simulink model "EMEAControls_BlockDiagram"  (R2016a)
settings: Solver=VariableStepAuto  StartTime=0.0  StopTime=10.0  RelTol=1e-3
undefined symbols (not defined in the file): ACTIVE, AIN03, AIN09, AIN13, AUX2, AUX2_FLOW_POT, BASE_ACTIVE, CD_AUX4_CONTROL_NEUTRAL, CD_AUX4_CRACKPOINT_CURRENT, CD_AUX4_MAX_FLOW_CURRENT, DIN08, DIN09, ENGINE_CRANKING, INIT_NORMAL, LEFT_HANDLE_BUTTON, LEFT_HANDLE_POT, MODE_AUX2_AUX4, MODE_AUX4_AUX2, MODE_AUX4_OFFSET, MODE_OFFSET_AUX4, MXSEC_AUX4_FLOW, NEUTRAL, OFFSET_SWITCH, RIGHT_HANDLE_POT, ROD_ACTIVE, SELECT_LEFT, SELECT_NEUTRAL, SELECT_RIGHT, SOC_LEFT, SOC_RIGHT
libraries: simulink x4, MX_Library x2
settings Model: Creator=aliebel  LastModifiedBy=aliebel

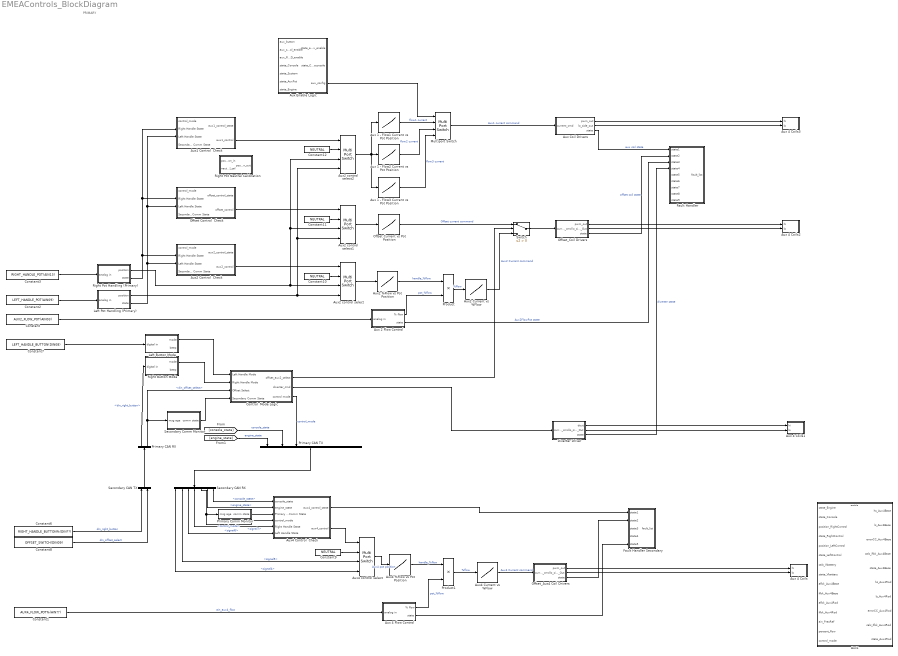
== system EMEAControls_BlockDiagram ==
  note: PRIMARY
  Aux 1 - Flow1 Current vs Pot Position : Lookup_n-D  NumberOfTableDimensions=1  BreakpointsForDimension1=[-5:5]  Table=tanh([-5:5])  InternalRulePriority=Speed  RndMeth=Simplest  InputSameDT=on
  Aux 1 - Flow2 Current vs Pot Position : Lookup_n-D  NumberOfTableDimensions=1  BreakpointsForDimension1=[-5:5]  Table=tanh([-5:5])  InternalRulePriority=Speed  RndMeth=Simplest  InputSameDT=on
  Aux 1 - Flow3 Current vs Pot Position : Lookup_n-D  NumberOfTableDimensions=1  BreakpointsForDimension1=[-5:5]  Table=tanh([-5:5])  InternalRulePriority=Speed  RndMeth=Simplest  InputSameDT=on
  Aux 2 Flow Control : Subsystem
  Aux 4 Coils : Subsystem
  Aux 4 Coils1 : Subsystem
  Aux 4 Coils2 : Subsystem
  Aux 4 Coils3 : Subsystem
  Aux 4 Flow Control : Subsystem
  Aux Coil Drivers : Subsystem
  Aux Enable Logic : Subsystem
  Aux1 : Subsystem
  Aux1 Control  Check : Subsystem
  Aux2 %Flow vs Pot Position : Lookup_n-D  NumberOfTableDimensions=1  BreakpointsForDimension1=[-5:5]  Table=tanh([-5:5])  InternalRulePriority=Speed  RndMeth=Simplest  InputSameDT=on
  Aux2 Current vs %Flow : Lookup_n-D  NumberOfTableDimensions=1  BreakpointsForDimension1=[-5:5]  Table=tanh([-5:5])  InternalRulePriority=Speed  RndMeth=Simplest  InputSameDT=on
  Aux2 Control  Check : Subsystem
  Aux2 control select : MultiPortSwitch
  Aux2 control select1 : MultiPortSwitch
  Aux2 control select2 : MultiPortSwitch
  Aux4 %Flow vs Pot Position : Lookup_n-D  NumberOfTableDimensions=1  BreakpointsForDimension1=[-5:5]  Table=tanh([-5:5])  InternalRulePriority=Speed  RndMeth=Simplest  InputSameDT=on
  Aux4 Current vs %Flow : Lookup_n-D  NumberOfTableDimensions=1  BreakpointsForDimension1=[-5:5]  Table=tanh([-5:5])  InternalRulePriority=Speed  RndMeth=Simplest  InputSameDT=on
  Aux4 Control  Check : Subsystem
  Aux4 control select : MultiPortSwitch
  Constant : Constant  Value=AUX2_FLOW_POT(AIN03)
  Constant1 : Constant  Value=AUX4_FLOW_POT%(AIN??)
  Constant{9..12} (4 alike) : Constant  Value=NEUTRAL
  Constant2 : Constant  Value=LEFT_HANDLE_POT(AIN09)
  Constant3 : Constant  Value=RIGHT_HANDLE_POT(AIN13)
  Constant6 : Constant  Value=RIGHT_HANDLE_BUTTON%(DIN??)
  Constant7 : Constant  Value=LEFT_HANDLE_BUTTON(DIN08)
  Constant8 : Constant  Value=OFFSET_SWITCH(DIN09)
  Control  Mode Logic : Subsystem
  Diverter Driver : Subsystem
  Fault Handler : Subsystem
  Fault Handler Secondary : Subsystem
  Left Button Mode : Subsystem
  Left Pot Handling (Primary) : Subsystem
  Multiport Switch : MultiPortSwitch
  Offset Current vs Pot Position : Lookup_n-D  NumberOfTableDimensions=1  BreakpointsForDimension1=[-5:5]  Table=tanh([-5:5])  InternalRulePriority=Speed  RndMeth=Simplest  InputSameDT=on
  Offset Control  Check : Subsystem
  Offset_Aux4 Coil Drivers : Subsystem
  Offset_Coil Drivers : Subsystem
  Primary CAN RX : BusSelector  OutputSignals=din_right_button,din_offset_select
  Primary CAN TX : BusCreator  Inputs=7
  Primary Comm Monitor : Subsystem
  Product : Product
  Product1 : Product
  Right Button Mode : Subsystem
  Right Pot Handling (Primary) : Subsystem
  Right Pot Neutral Calibration : Subsystem
  Secondary CAN RX : BusSelector  OutputSignals=signal4,signal5,signal6,signal7,control_mode,engine_state,console_state
  Secondary CAN TX : BusCreator  Inputs=2
  Secondary Comm Monitor : Subsystem
  Switch : Switch  Criteria=u2 > Threshold
  wires:
  Aux 1 - Flow1 Current vs Pot Position/1 -> Multiport Switch/2  "flow1 current"
  Multiport Switch/1 -> Aux Coil Drivers/1(current_cmd)  "Aux1 current command"
  Aux 1 - Flow2 Current vs Pot Position/1 -> Multiport Switch/3  "flow2 current"
  Aux 1 - Flow3 Current vs Pot Position/1 -> Multiport Switch/4  "flow3 current"
  Aux2 %Flow vs Pot Position/1 -> Product/1  "handle_%flow"
  Product/1 -> Aux2 Current vs %Flow/1  "%flow"
  Offset Current vs Pot Position/1 -> Switch/1  "Offset current command"
  Aux2 Current vs %Flow/1 -> Switch/3  "Aux2 Current command"
  Switch/1 -> Offset_Coil Drivers/1(current_cmd)
  Aux 2 Flow Control/1(% flow) -> Product/2  "pot_%flow"
  Aux4 %Flow vs Pot Position/1 -> Product1/1  "handle_%flow"
  Product1/1 -> Aux4 Current vs %Flow/1  "%flow"
  Aux4 Current vs %Flow/1 -> Offset_Aux4 Coil Drivers/1(current_cmd)  "Aux4 Current command"
  Aux 4 Flow Control/1(% flow) -> Product1/2  "pot_%flow"
  Aux Coil Drivers/3(state) -> Fault Handler/1(state1)  "aux coil state"
  Offset_Coil Drivers/3(state) -> Fault Handler/2(state2)  "offset coil state"
  Diverter Driver/3(state) -> Fault Handler/4(state4)  "diverter state"
  Aux 2 Flow Control/2(state) -> Fault Handler/3(state3)  "Aux2FlowPot state"
  Constant/1 -> Aux 2 Flow Control/1(analog in)
  Constant1/1 -> Aux 4 Flow Control/1(analog in)  "ain_aux4_flow"
  Primary CAN TX/1 -> Secondary CAN RX/1
  Secondary CAN TX/1 -> Primary CAN RX/1
  Constant7/1 -> Left Button Mode/1(digital in)
  Constant2/1 -> Left Pot Handling (Primary)/1(analog in)
  Constant3/1 -> Right Pot Handling (Primary)/1(analog in)
  Constant8/1 -> Secondary CAN TX/2  "din_offset_select"
  Constant6/1 -> Secondary CAN TX/1  "din_right_button"
  Primary Comm Monitor/1(comm state) -> Aux4 Control  Check/3(Primary Comm State)
  Secondary CAN RX/5 -> Primary Comm Monitor/1(msg age), Aux4 Control  Check/4(control_mode)  "<control_mode>"
  Aux4 Control  Check/1(aux4_control_state) -> Fault Handler Secondary/1(state1)
  Offset_Aux4 Coil Drivers/3(state) -> Fault Handler Secondary/2(state2)
  Aux4 Control  Check/2(aux4_control) -> Aux4 control select/1
  Constant9/1 -> Aux4 control select/2
  Aux4 control select/1 -> Aux4 %Flow vs Pot Position/1  "Aux4 pot position"
  Aux 4 Flow Control/2(state) -> Fault Handler Secondary/5(state5)
  Primary CAN RX/2 -> Control  Mode Logic/3(Offset Select), Secondary Comm Monitor/1(msg age)  "<din_offset_select>"
  Offset_Aux4 Coil Drivers/1(pwm_out) -> Aux 4 Coils/1("hi ")
  Offset_Aux4 Coil Drivers/2(lo_side_Out) -> Aux 4 Coils/2(lo)
  Primary CAN RX/1 -> Right Button Mode/1(digital in)  "<din_right_button>"
  Secondary Comm Monitor/1(comm state) -> Control  Mode Logic/4(Secondary Comm State)
  Right Button Mode/1(mode) -> Control  Mode Logic/2(Right Handle Mode)
  Left Button Mode/1(mode) -> Control  Mode Logic/1(Left Handle Mode)
  Control  Mode Logic/3(control mode) -> Primary CAN TX/3  "control_mode"
  Aux2 control select/1 -> Aux2 %Flow vs Pot Position/1
  Constant10/1 -> Aux2 control select/2
  Aux2 Control  Check/2(aux2_control) -> Aux2 control select/1
  Diverter Driver/1(dout) -> Aux 4 Coils1/1("hi ")
  Diverter Driver/2(lo_side_Out) -> Aux 4 Coils1/2(lo)
  Offset_Coil Drivers/1(pwm_out) -> Aux 4 Coils2/1("hi ")
  Offset_Coil Drivers/2(lo_side_Out) -> Aux 4 Coils2/2(lo)
  Aux Coil Drivers/1(pwm_out) -> Aux 4 Coils3/1("hi ")
  Aux Coil Drivers/2(lo_side_out) -> Aux 4 Coils3/2(lo)
  Constant11/1 -> Aux2 control select1/2
  Constant12/1 -> Aux2 control select2/2
  Aux2 control select2/1 -> Aux 1 - Flow1 Current vs Pot Position/1, Aux 1 - Flow3 Current vs Pot Position/1, Aux 1 - Flow2 Current vs Pot Position/1
  Aux2 control select1/1 -> Offset Current vs Pot Position/1
  Offset Control  Check/2(offset_control) -> Aux2 control select1/1
  Aux1 Control  Check/2(aux1_control) -> Aux2 control select2/1
  Left Pot Handling (Primary)/1(position) -> Aux2 control select2/4, Aux2 control select1/4, Aux2 control select/4
  Right Pot Handling (Primary)/1(position) -> Aux2 control select2/3, Aux2 control select1/3, Aux2 control select/3
  Right Pot Handling (Primary)/2(state) -> Offset Control  Check/2(Right Handle State), Aux1 Control  Check/2(Right Handle State), Aux2 Control  Check/2(Right Handle State)
  Left Pot Handling (Primary)/2(state) -> Aux1 Control  Check/3(Left Handle State), Offset Control  Check/3(Left Handle State), Aux2 Control  Check/3(Left Handle State)
  Control  Mode Logic/2(diverter_cmd) -> Diverter Driver/1(current_cmd)
  Control  Mode Logic/1(offset_aux2_select) -> Switch/2
  Aux Enable Logic/3(aux_config) -> Multiport Switch/1
  [console_state] -> Primary CAN TX/2  "console_state"
  [engine_state] -> Primary CAN TX/1  "engine_state"
  Secondary CAN RX/6 -> Aux4 Control  Check/2(engine_state)  "<engine_state>"
  Secondary CAN RX/7 -> Aux4 Control  Check/1(console_state)  "<console_state>"
  Secondary CAN RX/4 -> Aux4 Control  Check/5(Right Handle State)  "<signal7>"
  Secondary CAN RX/3 -> Aux4 Control  Check/6(Left Handle State)  "<signal6>"
  Secondary CAN RX/2 -> Aux4 control select/3  "<signal5>"
  Secondary CAN RX/1 -> Aux4 control select/4  "<signal4>"

== system EMEAControls_BlockDiagram/Aux 2 Flow Control ==
  analog in : Inport
  % flow : Outport
  state : Outport  Port=2
  wires:
  analog in/1 -> % flow/1

== system EMEAControls_BlockDiagram/Aux 4 Coils ==
  "hi " : Inport
  lo : Inport  Port=2

== system EMEAControls_BlockDiagram/Aux 4 Coils1 ==
  "hi " : Inport
  lo : Inport  Port=2

== system EMEAControls_BlockDiagram/Aux 4 Coils2 ==
  "hi " : Inport
  lo : Inport  Port=2

== system EMEAControls_BlockDiagram/Aux 4 Coils3 ==
  "hi " : Inport
  lo : Inport  Port=2

== system EMEAControls_BlockDiagram/Aux 4 Flow Control ==
  analog in : Inport
  % flow : Outport
  state : Outport  Port=2
  wires:
  analog in/1 -> % flow/1

== system EMEAControls_BlockDiagram/Aux Coil Drivers ==
  current_cmd : Inport
  pwm_out : Outport
  lo_side_out : Outport  Port=2
  state : Outport  Port=3
  wires:
  current_cmd/1 -> pwm_out/1

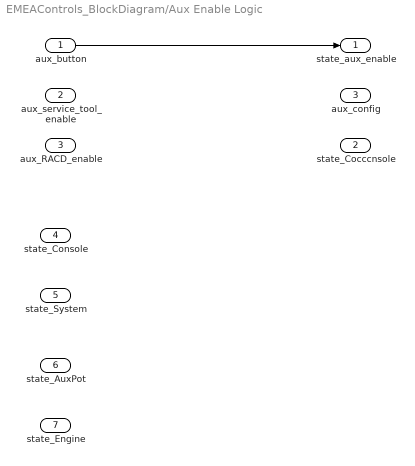
== system EMEAControls_BlockDiagram/Aux Enable Logic ==
  aux_button : Inport
  aux_service_tool_enable : Inport  Port=2
  aux_RACD_enable : Inport  Port=3
  state_Console : Inport  Port=4
  state_System : Inport  Port=5
  state_AuxPot : Inport  Port=6
  state_Engine : Inport  Port=7
  state_aux_enable : Outport
  state_Cocccnsole : Outport  Port=2
  aux_config : Outport  Port=3
  wires:
  aux_button/1 -> state_aux_enable/1

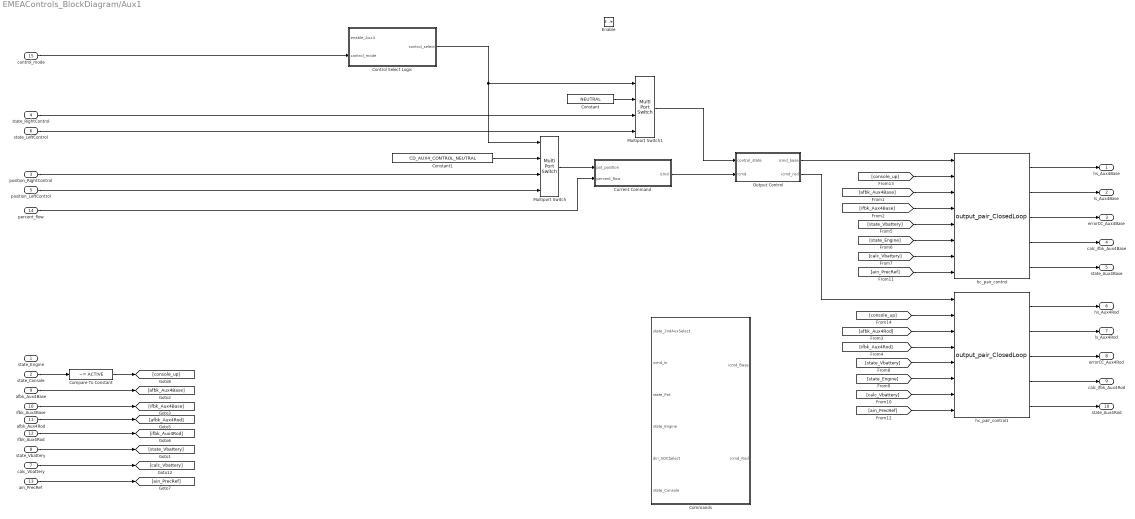
== system EMEAControls_BlockDiagram/Aux1 ==
  state_Engine : Inport
  state_Console : Inport  Port=2
  position_RightControl : Inport  Port=3
  state_RightControl : Inport  Port=4
  position_LeftControl : Inport  Port=5
  state_LeftControl : Inport  Port=6
  calc_Vbattery : Inport  Port=7
  state_Vbattery : Inport  Port=8
  afbk_Aux4Base : Inport  Port=9
  ifbk_Aux4Base : Inport  Port=10
  afbk_Aux4Rod : Inport  Port=11
  ifbk_Aux4Rod : Inport  Port=12
  ain_PrecRef : Inport  Port=13
  percent_flow : Inport  Port=14
  control_mode : Inport  Port=15
  Enable : EnablePort  StatesWhenEnabling=reset  PropagateVarSize=During execution
  Commands : Stateflow chart  TreatAsAtomicUnit=on
  Compare To Constant : simulink/Logic and Bit Operations/Compare To Constant  relop=~=  const=ACTIVE  OutDataTypeStr=boolean
  Constant : Constant  Value=NEUTRAL  OutDataTypeStr=uint8
  Constant1 : Constant  Value=CD_AUX4_CONTROL_NEUTRAL  OutDataTypeStr=uint8
  Control Select Logic : Truth Table  TreatAsAtomicUnit=on
  Current Command : Subsystem
  Multiport Switch : MultiPortSwitch
  Multiport Switch1 : MultiPortSwitch
  Output Control : Subsystem
  hc_pair_control : MX_Library/output_pair_ClosedLoop  AFBK_GAIN=CD_AUX4_AFBK_GAIN  IFBK_GAIN=CD_AUX4_IFBK_GAIN  OPEN_DB_CNT=CD_AUX4_DEBOUNCE_OPEN_CIRCUIT  STG_DB_CNT=CD_AUX4_DEBOUNCE_SHORT_TO_GROUND  OSTG_DB_CNT=CD_AUX4_DEBOUNCE_SHORT_TO_GROUND  STB_DB_CNT=CD_AUX4_DEBOUNCE_SHORT_TO_BATTERY  OC_DB_CNT=CD_AUX4_DEBOUNCE_OVERCURRENT  IFBK_MAX=CD_AUX4_OVERCURRENT  NZ_IFBK=CD_AUX4_NON_ZERO_CURRENT  NZ_DUTY=CD_AUX4_NON_ZERO_DUTY  KP=CD_AUX4_KP  KI=CD_AUX4_KI  BIDIRECTIONAL_CTRL=NON_FUNCTIONAL
  hc_pair_control1 : MX_Library/output_pair_ClosedLoop  AFBK_GAIN=CD_AUX4_AFBK_GAIN  IFBK_GAIN=CD_AUX4_IFBK_GAIN  OPEN_DB_CNT=CD_AUX4_DEBOUNCE_OPEN_CIRCUIT  STG_DB_CNT=CD_AUX4_DEBOUNCE_SHORT_TO_GROUND  OSTG_DB_CNT=CD_AUX4_DEBOUNCE_SHORT_TO_GROUND  STB_DB_CNT=CD_AUX4_DEBOUNCE_SHORT_TO_BATTERY  OC_DB_CNT=CD_AUX4_DEBOUNCE_OVERCURRENT  IFBK_MAX=CD_AUX4_OVERCURRENT  NZ_IFBK=CD_AUX4_NON_ZERO_CURRENT  NZ_DUTY=CD_AUX4_NON_ZERO_DUTY  KP=CD_AUX4_KP  KI=CD_AUX4_KI  BIDIRECTIONAL_CTRL=NON_FUNCTIONAL
  hs_Aux4Base : Outport  OutputWhenDisabled=reset  InitialOutput=[0]
  ls_Aux4Base : Outport  Port=2  OutputWhenDisabled=reset  InitialOutput=[0]
  errorCC_Aux4Base : Outport  Port=3  OutputWhenDisabled=reset  InitialOutput=[0]
  calc_ifbk_Aux4Base : Outport  Port=4  OutputWhenDisabled=reset  InitialOutput=[0]
  state_Aux4Base : Outport  Port=5  OutputWhenDisabled=reset  InitialOutput=[INIT_NORMAL]
  hs_Aux4Rod : Outport  Port=6  OutputWhenDisabled=reset  InitialOutput=[0]
  ls_Aux4Rod : Outport  Port=7  OutputWhenDisabled=reset  InitialOutput=[0]
  errorCC_Aux4Rod : Outport  Port=8  OutputWhenDisabled=reset  InitialOutput=[0]
  calc_ifbk_Aux4Rod : Outport  Port=9  OutputWhenDisabled=reset  InitialOutput=[0]
  state_Aux4Rod : Outport  Port=10  OutputWhenDisabled=reset  InitialOutput=[INIT_NORMAL]
  wires:
  state_Console/1 -> Compare To Constant/1
  hc_pair_control/1 -> hs_Aux4Base/1
  hc_pair_control/2 -> ls_Aux4Base/1
  hc_pair_control/3 -> errorCC_Aux4Base/1
  hc_pair_control/4 -> calc_ifbk_Aux4Base/1
  hc_pair_control1/1 -> hs_Aux4Rod/1
  hc_pair_control1/2 -> ls_Aux4Rod/1
  hc_pair_control1/3 -> errorCC_Aux4Rod/1
  hc_pair_control1/4 -> calc_ifbk_Aux4Rod/1
  afbk_Aux4Base/1 -> [afbk_Aux4Base]
  state_Vbattery/1 -> [state_Vbattery]
  afbk_Aux4Rod/1 -> [afbk_Aux4Rod]
  ifbk_Aux4Rod/1 -> [ifbk_Aux4Rod]
  calc_Vbattery/1 -> [calc_Vbattery]
  ifbk_Aux4Base/1 -> [ifbk_Aux4Base]
  hc_pair_control1/5 -> state_Aux4Rod/1
  hc_pair_control/5 -> state_Aux4Base/1
  [afbk_Aux4Base] -> hc_pair_control/3
  [ifbk_Aux4Base] -> hc_pair_control/4
  [state_Vbattery] -> hc_pair_control/5
  [state_Engine] -> hc_pair_control/6
  [calc_Vbattery] -> hc_pair_control/7
  [afbk_Aux4Rod] -> hc_pair_control1/3
  [ifbk_Aux4Rod] -> hc_pair_control1/4
  [state_Vbattery] -> hc_pair_control1/5
  [state_Engine] -> hc_pair_control1/6
  [calc_Vbattery] -> hc_pair_control1/7
  [ain_PrecRef] -> hc_pair_control1/8
  [ain_PrecRef] -> hc_pair_control/8
  ain_PrecRef/1 -> [ain_PrecRef]
  Compare To Constant/1 -> [console_up]
  [console_up] -> hc_pair_control/2
  [console_up] -> hc_pair_control1/2
  percent_flow/1 -> Current Command/2(percent_flow)
  Output Control/1(icmd_base) -> hc_pair_control/1
  Output Control/2(icmd_rod) -> hc_pair_control1/1
  Current Command/1(icmd) -> Output Control/2(icmd)
  Control Select Logic/1(control_select) -> Multiport Switch/1, Multiport Switch1/1
  Multiport Switch/1 -> Current Command/1(pot_position)
  Multiport Switch1/1 -> Output Control/1(control_state)
  position_RightControl/1 -> Multiport Switch/3
  position_LeftControl/1 -> Multiport Switch/4
  state_RightControl/1 -> Multiport Switch1/3
  state_LeftControl/1 -> Multiport Switch1/4
  control_mode/1 -> Control Select Logic/2(control_mode)
  Constant/1 -> Multiport Switch1/2
  Constant1/1 -> Multiport Switch/2

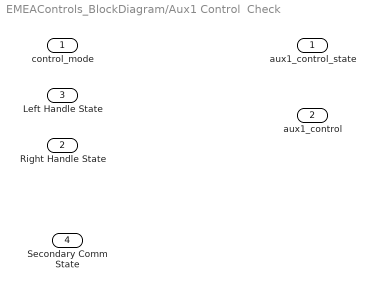
== system EMEAControls_BlockDiagram/Aux1 Control  Check ==
  control_mode : Inport
  Right Handle State : Inport  Port=2
  Left Handle State : Inport  Port=3
  Secondary Comm State : Inport  Port=4
  aux1_control_state : Outport
  aux1_control : Outport  Port=2

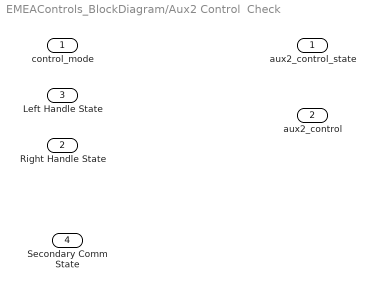
== system EMEAControls_BlockDiagram/Aux2 Control  Check ==
  control_mode : Inport
  Right Handle State : Inport  Port=2
  Left Handle State : Inport  Port=3
  Secondary Comm State : Inport  Port=4
  aux2_control_state : Outport
  aux2_control : Outport  Port=2

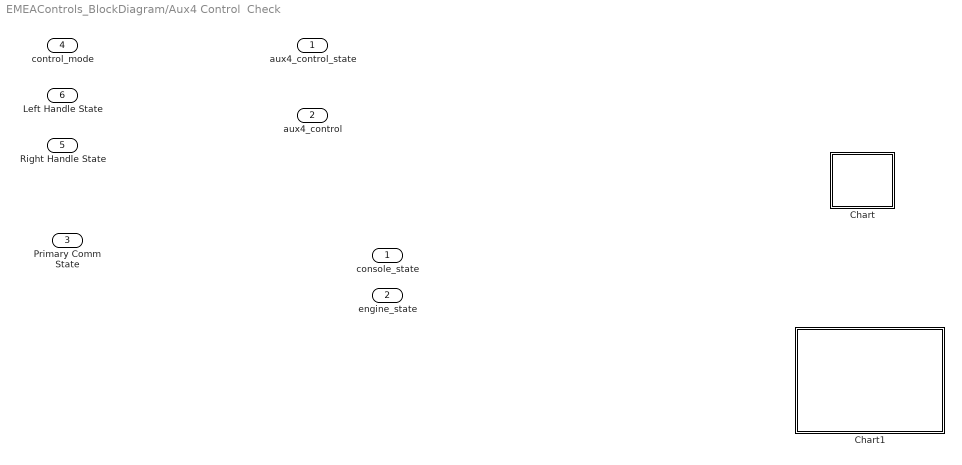
== system EMEAControls_BlockDiagram/Aux4 Control  Check ==
  console_state : Inport
  engine_state : Inport  Port=2
  Primary Comm State : Inport  Port=3
  control_mode : Inport  Port=4
  Right Handle State : Inport  Port=5
  Left Handle State : Inport  Port=6
  Chart : Stateflow chart  TreatAsAtomicUnit=on
  Chart1 : Stateflow chart  TreatAsAtomicUnit=on
  aux4_control_state : Outport
  aux4_control : Outport  Port=2

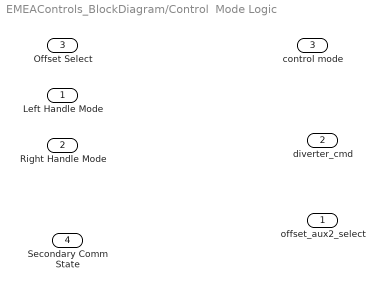
== system EMEAControls_BlockDiagram/Control  Mode Logic ==
  Left Handle Mode : Inport
  Right Handle Mode : Inport  Port=2
  Offset Select : Inport  Port=3
  Secondary Comm State : Inport  Port=4
  offset_aux2_select : Outport
  diverter_cmd : Outport  Port=2
  control mode : Outport  Port=3

== system EMEAControls_BlockDiagram/Diverter Driver ==
  current_cmd : Inport
  dout : Outport
  lo_side_Out : Outport  Port=2
  state : Outport  Port=3
  wires:
  current_cmd/1 -> dout/1

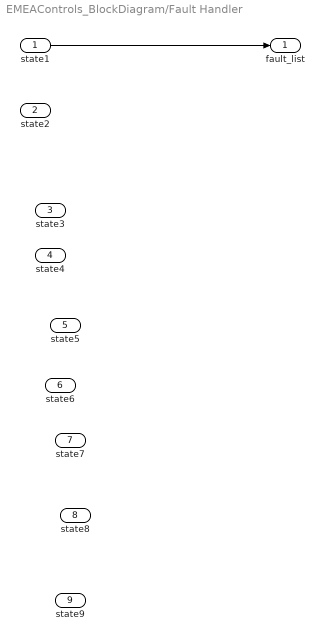
== system EMEAControls_BlockDiagram/Fault Handler ==
  state1 : Inport
  state2 : Inport  Port=2
  state3 : Inport  Port=3
  state4 : Inport  Port=4
  state5 : Inport  Port=5
  state6 : Inport  Port=6
  state7 : Inport  Port=7
  state8 : Inport  Port=8
  state9 : Inport  Port=9
  fault_list : Outport
  wires:
  state1/1 -> fault_list/1

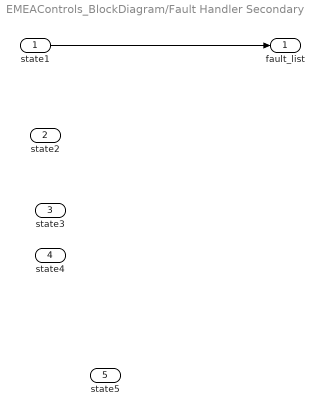
== system EMEAControls_BlockDiagram/Fault Handler Secondary ==
  state1 : Inport
  state2 : Inport  Port=2
  state3 : Inport  Port=3
  state4 : Inport  Port=4
  state5 : Inport  Port=5
  fault_list : Outport
  wires:
  state1/1 -> fault_list/1

== system EMEAControls_BlockDiagram/Left Button Mode ==
  digital in : Inport
  mode : Outport
  beep : Outport  Port=2
  wires:
  digital in/1 -> mode/1

== system EMEAControls_BlockDiagram/Left Pot Handling (Primary) ==
  analog in : Inport
  position : Outport
  state : Outport  Port=2
  wires:
  analog in/1 -> position/1

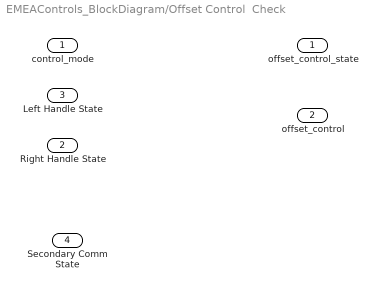
== system EMEAControls_BlockDiagram/Offset Control  Check ==
  control_mode : Inport
  Right Handle State : Inport  Port=2
  Left Handle State : Inport  Port=3
  Secondary Comm State : Inport  Port=4
  offset_control_state : Outport
  offset_control : Outport  Port=2

== system EMEAControls_BlockDiagram/Offset_Aux4 Coil Drivers ==
  current_cmd : Inport
  pwm_out : Outport
  lo_side_Out : Outport  Port=2
  state : Outport  Port=3
  wires:
  current_cmd/1 -> pwm_out/1

== system EMEAControls_BlockDiagram/Offset_Coil Drivers ==
  current_cmd : Inport
  pwm_out : Outport
  lo_side_Out : Outport  Port=2
  state : Outport  Port=3
  wires:
  current_cmd/1 -> pwm_out/1

== system EMEAControls_BlockDiagram/Primary Comm Monitor ==
  msg age : Inport
  comm state : Outport
  wires:
  msg age/1 -> comm state/1

== system EMEAControls_BlockDiagram/Right Button Mode ==
  digital in : Inport
  mode : Outport
  beep : Outport  Port=2
  wires:
  digital in/1 -> mode/1

== system EMEAControls_BlockDiagram/Right Pot Handling (Primary) ==
  analog in : Inport
  position : Outport
  state : Outport  Port=2
  wires:
  analog in/1 -> position/1

== system EMEAControls_BlockDiagram/Right Pot Neutral Calibration ==
  position_in : Inport
  neutral_cal : Inport  Port=2
  position_out : Outport
  wires:
  position_in/1 -> position_out/1

== system EMEAControls_BlockDiagram/Secondary Comm Monitor ==
  msg age : Inport
  comm state : Outport
  wires:
  msg age/1 -> comm state/1

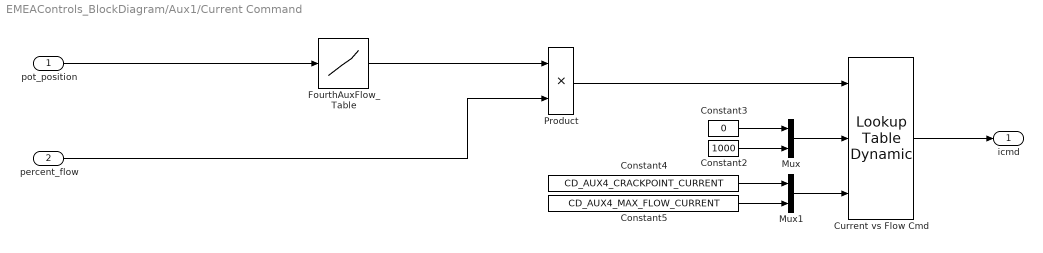
== system EMEAControls_BlockDiagram/Aux1/Current Command ==
  pot_position : Inport
  percent_flow : Inport  Port=2
  Constant2 : Constant  Value=1000  OutDataTypeStr=uint16
  Constant3 : Constant  Value=0  OutDataTypeStr=uint16
  Constant4 : Constant  Value=CD_AUX4_CRACKPOINT_CURRENT  OutDataTypeStr=fixdt(0,16,12)
  Constant5 : Constant  Value=CD_AUX4_MAX_FLOW_CURRENT  OutDataTypeStr=fixdt(0,16,12)
  Current vs Flow Cmd : simulink/Lookup Tables/Lookup Table Dynamic  LookUpMeth=Interpolation-Use End Values  OutDataTypeStr=fixdt('double')  OutputDataTypeScalingMode=Specify via dialog  OutDataType=fixdt('double')  OutScaling=2^-10  DoSatur=off
  FourthAuxFlow_Table : Lookup  InputValues=[0:20:1000]  Table=MXSEC_AUX4_FLOW  LookUpMeth=Interpolation-Use End Values  OutDataTypeStr=fixdt(0,16,12)  SaturateOnIntegerOverflow=on
      settings: AttributesFormatString=input = %<InputValues>\noutput = %<OutputValues>
  Mux : Mux  Inputs=2
  Mux1 : Mux  Inputs=2
  Product : Product
  icmd : Outport
  wires:
  Mux1/1 -> Current vs Flow Cmd/3
  Constant5/1 -> Mux1/2
  Mux/1 -> Current vs Flow Cmd/2
  Product/1 -> Current vs Flow Cmd/1
  Constant2/1 -> Mux/2
  percent_flow/1 -> Product/2
  Constant3/1 -> Mux/1
  Constant4/1 -> Mux1/1
  Current vs Flow Cmd/1 -> icmd/1
  pot_position/1 -> FourthAuxFlow_Table/1
  FourthAuxFlow_Table/1 -> Product/1

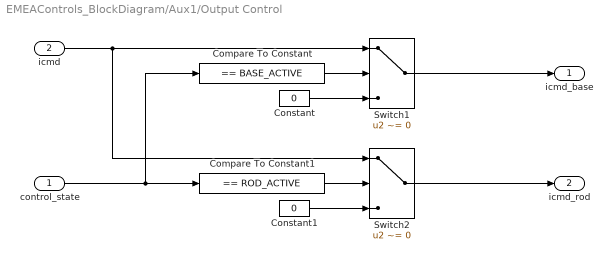
== system EMEAControls_BlockDiagram/Aux1/Output Control ==
  control_state : Inport
  icmd : Inport  Port=2
  Compare To Constant : simulink/Logic and Bit Operations/Compare To Constant  relop===  const=BASE_ACTIVE  OutDataTypeStr=boolean
  Compare To Constant1 : simulink/Logic and Bit Operations/Compare To Constant  relop===  const=ROD_ACTIVE  OutDataTypeStr=boolean
  Constant : Constant  Value=0  OutDataTypeStr=fixdt(0,16,12)
  Constant1 : Constant  Value=0  OutDataTypeStr=fixdt(0,16,12)
  Switch1 : Switch  Criteria=u2 ~= 0
  Switch2 : Switch  Criteria=u2 ~= 0
  icmd_base : Outport
  icmd_rod : Outport  Port=2
  wires:
  Compare To Constant/1 -> Switch1/2
  Constant/1 -> Switch1/3
  icmd/1 -> Switch1/1, Switch2/1
  Switch2/1 -> icmd_rod/1
  Switch1/1 -> icmd_base/1
  Constant1/1 -> Switch2/3
  Compare To Constant1/1 -> Switch2/2
  control_state/1 -> Compare To Constant/1, Compare To Constant1/1

== stateflow chart EMEAControls_BlockDiagram/Aux4 Control  Check/Chart1 ==
  state INACTIVE
  note: Check for pot neutral under following conditions:
      | Any mode change
      | Console lowered
      | Engine Cranking
      | Aux Enable Pressed??
  state AUX4_ON_LEFT
    state MODE_AUX4_OFFSET
    state MODE_AUX4_AUX1
  state AUX4_ON_RIGHT
    state MODE_OFFSET_AUX4
    state MODE_AUX2_AUX4
  state ?
  (default) -> INACTIVE
  INACTIVE -> AUX4_ON_RIGHT
  AUX4_ON_RIGHT -> INACTIVE

== stateflow chart EMEAControls_BlockDiagram/Aux4 Control  Check/Chart ==
  state INACTIVE
  note: Check for pot neutral under following conditions:
      | Any mode change
      | Console lowered
      | Engine Cranking
      | Aux Enable Pressed??
  state AUX4_ON_LEFT
    state MODE_AUX4_OFFSET
    state MODE_AUX4_AUX1
  state AUX4_ON_RIGHT
    state MODE_OFFSET_AUX4
    state MODE_AUX2_AUX4
  (default) -> INACTIVE
  INACTIVE -> AUX4_ON_RIGHT
  AUX4_ON_RIGHT -> INACTIVE

== stateflow chart EMEAControls_BlockDiagram/Aux1/Commands ==
  state Disabled
  state Active
    state Neutral
      en:
      icmd_Base = 0;
      icmd_Rod = 0;
    state RodActive
      en:
      icmd_Base = 0;
      icmd_Rod = icmd_In;
      du:
      icmd_Rod = icmd_In;
    state BaseActive
      en:
      icmd_Rod = 0;
      icmd_Base = icmd_In;
      du:
      icmd_Base = icmd_In;
    (default) -> Neutral
    Neutral -> RodActive [order 1] : [state_Pot == ROD_ACTIVE]
    BaseActive -> Neutral [order 1] : [state_Pot == NEUTRAL]
    Neutral -> BaseActive [order 2] : [state_Pot == BASE_ACTIVE]
    RodActive -> Neutral [order 1] : [state_Pot == NEUTRAL]
    BaseActive -> RodActive [order 2] : [state_Pot == ROD_ACTIVE]
    RodActive -> BaseActive [order 2] : [state_Pot == BASE_ACTIVE]
  (default) -> Disabled
  Disabled -> Active : [state_Console == ACTIVE &&...
      |  state_Engine != ENGINE_CRANKING]
  Active -> Disabled : [state_Console != ACTIVE ||...
      |  state_Engine == ENGINE_CRANKING ||...
      |  (din_SOCSelect == SOC_LEFT &&...
      |      state_2ndAuxSelect != AUX2)]
  data: state_2ndAuxSelect input uint8; icmd_In input fixdt(0,16,12); state_Pot input uint8; state_Engine input uint8; ENGINE_CRANKING parameter uint8; icmd_Base output fixdt(0,16,12); BASE_ACTIVE parameter uint8; NEUTRAL parameter uint8; ROD_ACTIVE parameter uint8; ACTIVE parameter uint8; icmd_Rod output fixdt(0,16,12); din_SOCSelect input boolean; state_Console input uint8; SOC_RIGHT parameter uint8; SOC_LEFT parameter uint8; AUX2 parameter uint8

== matlab function EMEAControls_BlockDiagram/Aux1/Control Select Logic ==
  data: enable_Aux4 input boolean; control_select output uint8; control_mode input uint8; MODE_OFFSET_AUX4 parameter uint8; MODE_AUX2_AUX4 parameter uint8; MODE_AUX4_OFFSET parameter uint8; MODE_AUX4_AUX2 parameter uint8; SELECT_LEFT parameter uint8; SELECT_RIGHT parameter uint8; SELECT_NEUTRAL parameter uint8
function control_select = fcn(enable_Aux4, control_mode, MODE_OFFSET_AUX4, MODE_AUX2_AUX4, MODE_AUX4_OFFSET, MODE_AUX4_AUX2, SELECT_LEFT, SELECT_RIGHT, SELECT_NEUTRAL)

aVarTruthTableCondition_1 = false;
aVarTruthTableCondition_2 = false;
aVarTruthTableCondition_3 = false;


% Aux4 Enabled

aVarTruthTableCondition_1 = logical(enable_Aux4 == 1;);

% Aux4 On Right

aVarTruthTableCondition_2 = logical(control_mode == MODE_OFFSET_AUX4 || control_mode == MODE_AUX2_AUX4);

% Aux4 On Left

aVarTruthTableCondition_3 = logical(control_mode == MODE_AUX4_OFFSET || control_mode == MODE_AUX4_AUX2);

if (aVarTruthTableCondition_1 && aVarTruthTableCondition_2 && ~aVarTruthTableCondition_3)
    aFcnTruthTableAction_1();
elseif (aVarTruthTableCondition_1 && ~aVarTruthTableCondition_2 && aVarTruthTableCondition_3)
    aFcnTruthTableAction_2();
else % Default
    aFcnTruthTableAction_3();
end

function aFcnTruthTableAction_1()

% Aux 4 on Right

control_select = SELECT_RIGHT;

function aFcnTruthTableAction_2()

% Aux 4 on Left

control_select = SELECT_LEFT;

function aFcnTruthTableAction_3()

% Aux 4 in Neutral

control_select = SELECT_NEUTRAL;
